simulink model "controllo_SS_no_obs2023bL_v2"  (R2023b)
settings: Solver=VariableStepAuto  StartTime=0.0  StopTime=20.0  RelTol=1e-3
values from neighbouring files (symbols this model uses):
  Ken_eta = Ken(:, n+1:end)    [LQ_KF_L.m]    (also in LQ_Luenberger_L.m = K(:, 4))
  Ken_x = Ken(:, 1:n)    [LQ_KF_L.m]    (also in LQ_Luenberger_L.m = K(:, 1:3))
undefined symbols (not defined in the file or in its folder): Lc, Rtot
libraries: simulink x1
settings Model: Creator=Pronto all'uso  LastModifiedBy=lollo

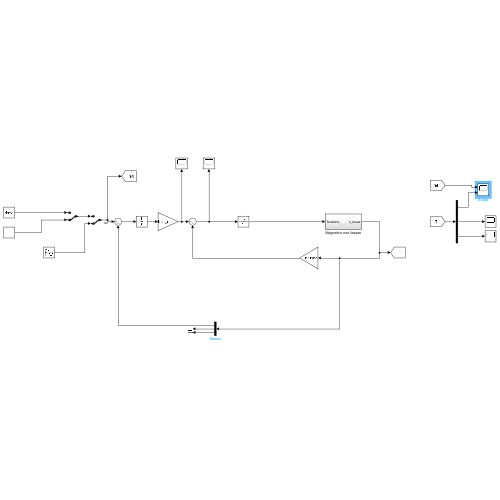
[thumbnail: Simulink's stored preview of the top-level diagram]
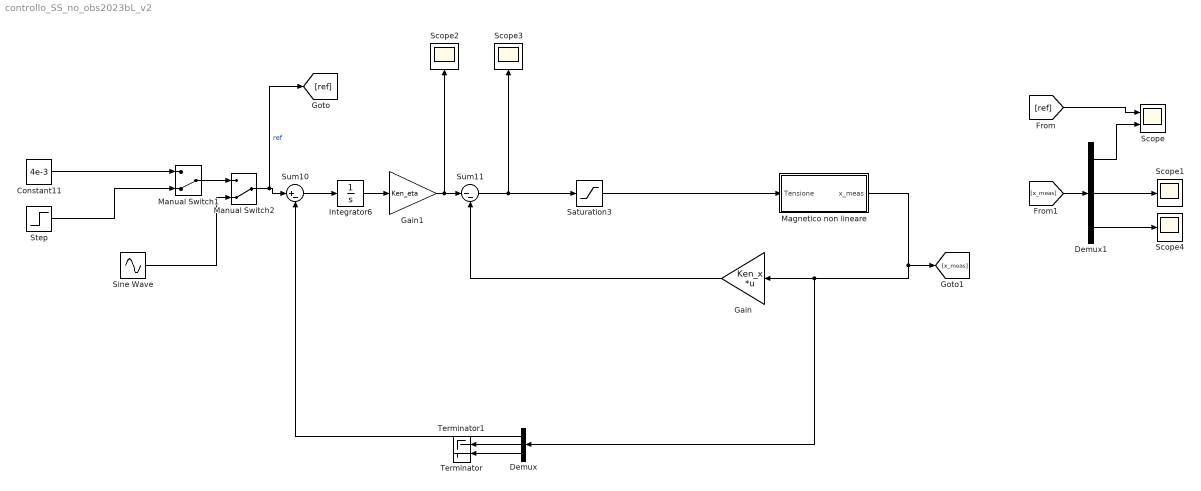
== system controllo_SS_no_obs2023bL_v2 ==
  Constant11 : Constant  Value=4e-3
  Demux : Demux  Outputs=3
  Demux1 : Demux  Outputs=3
  Gain : Gain  Gain=Ken_x  Multiplication=Matrix(K*u) (u vector)
  Gain1 : Gain  Gain=Ken_eta
  Integrator6 : Integrator
  Magnetico non lineare : Subsystem
  Manual Switch1 : ManualSwitch  CurrentSetting=0
  Manual Switch2 : ManualSwitch  CurrentSetting=0
  Saturation3 : Saturate  UpperLimit=24  LowerLimit=-24
  Scope : Scope  NumInputPorts=2
  Scope{1..4} (4 alike) : Scope
  Sine Wave : Sin  Amplitude=0.001  Bias=0.004  Frequency=4  SampleTime=0
  Step : Step  After=0.004  SampleTime=0
  Sum10 : Sum  Inputs=|+-
  Sum11 : Sum  Inputs=|--
  Terminator : Terminator
  Terminator1 : Terminator
  wires:
  Sum11/1 -> Saturation3/1, Scope3/1
  Integrator6/1 -> Gain1/1
  Manual Switch1/1 -> Manual Switch2/1
  Sine Wave/1 -> Manual Switch2/2
  Manual Switch2/1 -> [ref], Sum10/1  "ref"
  Gain1/1 -> Sum11/1, Scope2/1
  Sum10/1 -> Integrator6/1
  Constant11/1 -> Manual Switch1/1
  Step/1 -> Manual Switch1/2
  Magnetico non lineare/1(x_meas) -> [x_meas], Demux/1, Gain/1
  Gain/1 -> Sum11/2
  Saturation3/1 -> Magnetico non lineare/1(Tensione)
  Demux/2 -> Terminator1/1
  Demux/3 -> Terminator/1
  Demux/1 -> Sum10/2
  [x_meas] -> Demux1/1
  [ref] -> Scope/1
  Demux1/1 -> Scope/2
  Demux1/3 -> Scope4/1
  Demux1/2 -> Scope1/1

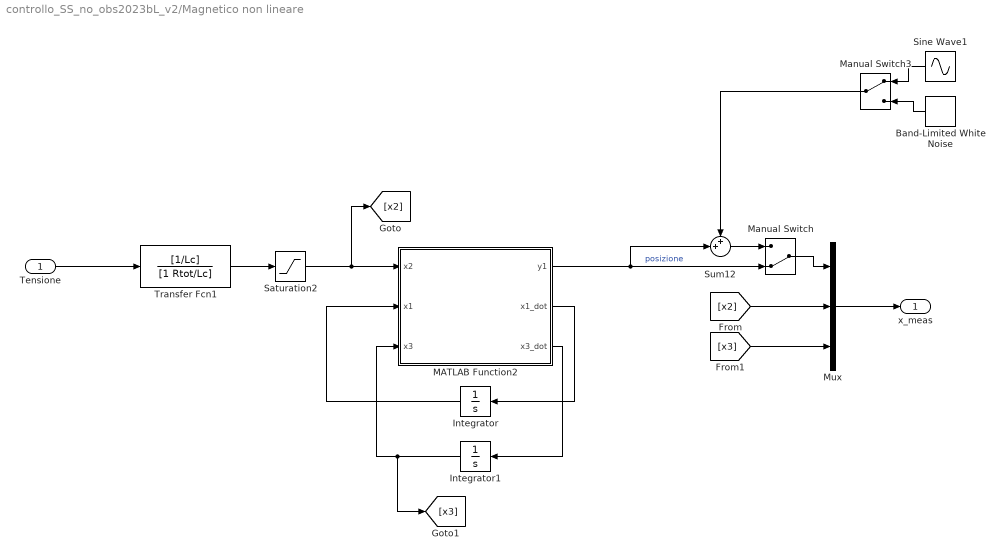
== system controllo_SS_no_obs2023bL_v2/Magnetico non lineare ==
  Tensione : Inport
  Band-Limited White Noise : simulink/Sources/Band-Limited White Noise  Cov=[8.9934e-11*0.002]  Ts=0.002  seed=[23341]
  Integrator : Integrator
  Integrator1 : Integrator
  MATLAB Function2 : MATLAB Function  TreatAsAtomicUnit=on
  Manual Switch : ManualSwitch  CurrentSetting=0
  Manual Switch3 : ManualSwitch
  Mux : Mux  Inputs=3
  Saturation2 : Saturate  UpperLimit=3  LowerLimit=0
  Sine Wave1 : Sin  Amplitude=0.00001  Frequency=50  SampleTime=0.002
  Sum12 : Sum  Inputs=++|
  Transfer Fcn1 : TransferFcn  Numerator=[1/Lc]  Denominator=[1 Rtot/Lc]
  x_meas : Outport
  wires:
  MATLAB Function2/1(y1) -> Manual Switch/2, Sum12/2  "posizione"
  MATLAB Function2/2(x1_dot) -> Integrator/1
  Integrator/1 -> MATLAB Function2/2(x1)
  MATLAB Function2/3(x3_dot) -> Integrator1/1
  Integrator1/1 -> [x3], MATLAB Function2/3(x3)
  Transfer Fcn1/1 -> Saturation2/1
  Saturation2/1 -> [x2], MATLAB Function2/1(x2)
  Tensione/1 -> Transfer Fcn1/1
  [x2] -> Mux/2
  [x3] -> Mux/3
  Mux/1 -> x_meas/1
  Band-Limited White Noise/1 -> Manual Switch3/2
  Sine Wave1/1 -> Manual Switch3/1
  Manual Switch3/1 -> Sum12/1
  Sum12/1 -> Manual Switch/1
  Manual Switch/1 -> Mux/1

== matlab function controllo_SS_no_obs2023bL_v2/Magnetico non lineare/MATLAB Function2 ==
  data: y1 output; x2 input; x1_dot output; x1 input; x3 input; x3_dot output
function [y1,x1_dot, x3_dot] = fcn(x2, x1, x3)
    m = 0.0657;
    g = 9.81;
    k_mag = 2.4405e-05;
    Rtot = 9.7585;
    Lc = 0.3708;
    y0 = 0.012;
    
    x1_dot = x3;
    if x1 < y0
        x3_dot = (k_mag/m)*(x2/(y0-x1))^2 - g;
    else
        x1 = 0.012;
        x3_dot = 0;
        x3 = 0;
    end

    
    % condizioni
    if x1 <=0 && x3_dot < 0
        x1 = 0;
        x3 = 0;
        x3_dot = 0;
    end
y1 = x1;
